simulink model "do178b_dhc2_rev_new"  (R2021b)
settings: Solver=ode23  StartTime=0.0  StopTime=25  MaxStep=1/40  RelTol=1e-2  AbsTol=1e-3  EnableMultiTasking=on
PreLoadFcn:
  | load asbdhc2_init;
  | Autopilot_bus;
model workspace (MAT data in the model file):
  ALT_Mode = [0 0 0 0 0 0 0 0 0 0 0 0 ... (1001 elements, 1001x1)]
  ALT_Ref = [991.703720962 991.703720962 991.703720962 991.703720962 991.703720962 991.703720962 991.703720962 991.703720962 991.703720962 991.703720962 991.703720962 991.703720962 ... (1001 elements, 1001x1)]
  AP_Eng = [1 1 1 1 1 1 1 1 1 1 1 1 ... (1001 elements, 1001x1)]
  AilCmdv = [0; 0; 0]
  Ail_cmd : timeseries (value not decoded)
  FR = [0; 0]
  Ft = [0 0.333333333333 0.333333333333 0.333333333333 0.333333333333 0.333333333333 0.333333333333 0.333333333333 0.333333333333 0.333333333333 0.333333333333 0.333333333333 ... (1001 elements, 1001x1)]
  HDG_Mode = [0 0 0 0 0 0 0 0 0 0 0 0 ... (1001 elements, 1001x1)]
  HDG_Ref = [29.7066688805 29.7066688805 29.7066688805 29.7066688805 29.7066688805 29.7066688805 29.7066688805 29.7066688805 29.7066688805 29.7066688805 29.7066688805 29.7066688805 ... (1001 elements, 1001x1)]
  InputSize = 2
  N = 37
  PhiRefv = [0; 0; 0]
  Phi_Ref : timeseries (value not decoded)
  Phiv = [0; 0; 0]
  Pwheel = [2.59796598511 2.59796598511 2.59796598511 2.59796598511 2.59796598511 2.59796598511 2.59796598511 2.59796598511 2.59796598511 2.59796598511 2.59796598511 2.59796598511 ... (1001 elements, 1001x1)]
  Roll_Mode = [1 1 1 1 1 1 1 1 1 1 1 1 ... (1001 elements, 1001x1)]
  TimeSteps = 1001
  Tkv = [0; 0; 0]
  TurnK = [-15.9132354515 -15.9132354515 -15.9132354515 -15.9132354515 -15.9132354515 -15.9132354515 -15.9132354515 -15.9132354515 -15.9132354515 -15.9132354515 -15.9132354515 -15.9132354515 ... (1001 elements, 1001x1)]
  X = [1 1 1 0 0 0 0 0 1 81.536789931 -1.01532751936 38.5971284353 ... (24 elements, 1x24)]
  a = 0.726747501556
  a1 = [0.30275909672 0.30275909672 0.30275909672 0.30275909672 0.30275909672 0.30275909672 0.30275909672 0.30275909672 0.30275909672 0.30275909672 0.30275909672 0.30275909672 ... (1001 elements, 1x1001)]
  apin : object (value not decoded)
  apsin : time (value not decoded)
  curPath = 'C:\Python-Workspace\thesis\new FSE2019\ModeTestingData\Problems'
  d = 25
  hws : Simulink.ModelWorkspace (value not decoded)
  i = 9
  inertial : object (value not decoded)
  j = 8
  list : object (value not decoded)
  modelpath = 'C:\Python-Workspace\thesis\new FSE2019\Benchmark\Simulink Models\autopilot\aprevised\'
  models : object (value not decoded)
  n = 1
  nbrInputs = 8
  req = 'R12.1'
  rollOut = []
  simOut : Simulink.SimulationOutput (value not decoded)
  t = [0 0.025 0.05 0.075 0.1 0.125 0.15 0.175 0.2 0.225 0.25 0.275 ... (1001 elements, 1x1001)]
undefined symbols (not defined in the file): beaver_b, beaver_c, beaver_init_p, beaver_init_pitch, beaver_init_q, beaver_init_r, beaver_init_roll, beaver_mass, Cl0, Cl_alpha2_dpt, Cl_beta, Cl_da, Cl_da_alpha, Cl_dr, Cl_p, Cl_r, Cm0, Cm_alpha, Cm_alpha2, Cm_beta2, Cm_de, Cm_df, Cm_dpt, Cm_q, Cm_r, Cn0, Cn_beta, Cn_beta3, Cn_da, Cn_dpt3, Cn_dr, Cn_p, Cn_q, Cn_r, Cx0, Cx_alpha, Cx_alpha2, Cx_alpha3, Cx_df, Cx_df_alpha, Cx_dpt, Cx_dpt2_alpha, Cx_dr, Cx_q, Cy0, Cy_beta, Cy_da, Cy_dr, Cy_dr_alpha, Cy_p, Cy_r, Cz0, Cz_alpha, Cz_alpha3, Cz_de, Cz_de_beta, Cz_df, Cz_df_alpha, Cz_dpt, Cz_q ... (+9)
libraries: aerolibconvert2 x6, simulink x6, aerolibobsolete x5, aerolibasang x3, aerolibwind2 x3, aerolibadyn x1, aerolibatmos2 x1
(part 2 of 3)

== system do178b_dhc2_rev_new/Air Data Sensor ==
  note: Air Data Sensor
  AC Bus : Inport
  Bus Creator : BusCreator  Inputs=5
  Bus Selector : BusSelector  OutputSignals=Hdot,Ve,xyh
  Length Conversion : aerolibconvert2/Length Conversion  IU=m  OU=ft
  Rate Transition1 : RateTransition  OutPortSampleTime=1/40
  Rate Transition2 : RateTransition  InitialCondition=2202  OutPortSampleTime=1/40
  Rate Transition3 : RateTransition  InitialCondition=[44.54 2.714 5.836]  OutPortSampleTime=1/40
  Selector1 : Selector  InputPortWidth=3  IndexOptions=Index vector (dialog)  Indices=[3]  OutputSizes=1
  Velocity Conversion : aerolibconvert2/Velocity Conversion  IU=m/s  OU=ft/s
  Velocity Conversion1 : aerolibconvert2/Velocity Conversion  IU=m/s  OU=ft/s
  "alpha, beta, TAS" : aerolibasang/Incidence, Sideslip, & Airspeed
  Air Data : Outport  VectorParamsAs1DForOutWhenUnconnected=off
  wires:
  AC Bus/1 -> Bus Selector/1
  Bus Selector/1 -> Velocity Conversion/1  "<Hdot>"
  Bus Selector/2 -> Rate Transition3/1  "<Ve>"
  Bus Selector/3 -> Selector1/1  "<xyh>"
  Bus Creator/1 -> Air Data/1
  Rate Transition1/1 -> Bus Creator/1  "altRate"
  Selector1/1 -> Rate Transition2/1
  "alpha, beta, TAS"/1 -> Bus Creator/2  "alpha"
  "alpha, beta, TAS"/2 -> Bus Creator/3  "beta"
  "alpha, beta, TAS"/3 -> Bus Creator/4  "airspeed"
  Velocity Conversion/1 -> Rate Transition1/1
  Length Conversion/1 -> Bus Creator/5  "alt"
  Velocity Conversion1/1 -> "alpha, beta, TAS"/1
  Rate Transition3/1 -> Velocity Conversion1/1
  Rate Transition2/1 -> Length Conversion/1

== system do178b_dhc2_rev_new/Cockpit Controls ==
  Demux : Demux  Tag=STV Demux  Outputs=2
      settings: DisplayOption=none
  FromWs : FromWorkspace  Tag=STV FromWs  VariableName=tuvar
      SigBuilderData=|
      | common.afterFinalStr = 'Extrapolate'
      | common.sampleTime = 0
      | dataSet.timeRange = [0 10]
      | dataSet.name = 'Steady State Flight'
      | sbobj.Groups.Name = 'Steady State Flight'
      | sbobj.Groups.Signals(1).Name = 'Flap Handle'
      | sbobj.Groups.Signals(1).XData = [0 10]
      | sbobj.Groups.Signals(1).YData = [0 0]
      | sbobj.Groups.Signals(2).Name = 'Rudder Trim'
      | sbobj.Groups.Signals(2).XData = [0 10]
      | sbobj.Groups.Signals(2).YData = [0 0]
  Flap Handle : Outport  Tag=STV Outport  VectorParamsAs1DForOutWhenUnconnected=off
  Rudder Trim : Outport  Tag=STV Outport  Port=2  VectorParamsAs1DForOutWhenUnconnected=off
  wires:
  FromWs/1 -> Demux/1
  Demux/1 -> Flap Handle/1
  Demux/2 -> Rudder Trim/1

== system do178b_dhc2_rev_new/DeHavilland Beaver Airframe ==
  note: DeHavilland Beaver Airframe
  EnvirBus : Inport
  Pilot : Inport  Port=2
  Aircraft Dynamics : Subsystem
  Calculate Parameters : Subsystem
  ACBus : Outport  VectorParamsAs1DForOutWhenUnconnected=off
  wires:
  Pilot/1 -> Aircraft Dynamics/1(Pilot)
  Aircraft Dynamics/1(AC Bus) -> ACBus/1, Calculate Parameters/2(ACBus)
  EnvirBus/1 -> Aircraft Dynamics/2(EnvirBus), Calculate Parameters/1(EnvirBus)
  Calculate Parameters/1(FltParams) -> Aircraft Dynamics/3(FltParams)

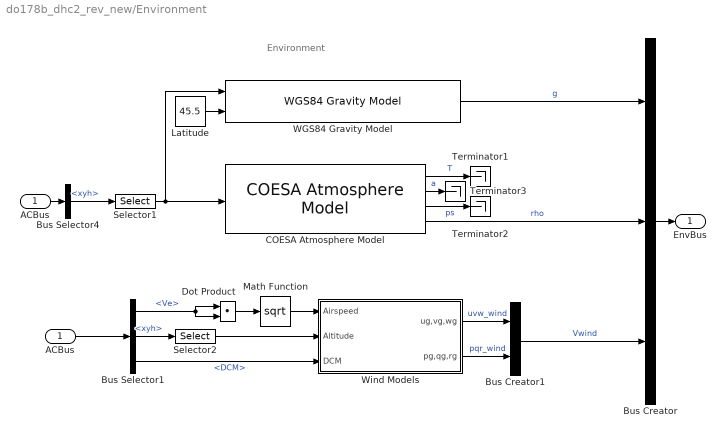
== system do178b_dhc2_rev_new/Environment ==
  note: Environment
  ACBus : Inport
  "ACBus " : InportShadow
  Bus Creator : BusCreator  Inputs=3
  Bus Creator1 : BusCreator  Inputs=2
  Bus Selector1 : BusSelector  OutputSignals=Ve,xyh,DCM
  Bus Selector4 : BusSelector  OutputSignals=xyh
  COESA Atmosphere Model : aerolibatmos2/COESA Atmosphere Model  units=Metric (MKS)  spec=1976 COESA-extended U.S. Standard Atmosphere  model=Profile  profile_var=High temperature  profile_percent=1%  profile_alt=5 km (16404 ft)  envelope_var=High temperature  envelope_percent=1%  action=Warning
  Dot Product : DotProduct  InputSameDT=on  OutDataTypeStr=Inherit: Inherit via internal rule
  Latitude : Constant  Value=45.5
  Math Function : Math  Operator=sqrt  SignedPower=on  SaturateOnIntegerOverflow=on
  Selector1 : Selector  InputPortWidth=3  IndexOptions=Index vector (dialog)  Indices=[3]  OutputSizes=1
  Selector2 : Selector  InputPortWidth=3  IndexOptions=Index vector (dialog)  Indices=[3]  OutputSizes=1
  Terminator1 : Terminator
  Terminator2 : Terminator
  Terminator3 : Terminator
  WGS84 Gravity Model : aerolibobsolete/WGS84 Gravity Model  model=WGS84 Taylor Series  units=Metric (MKS)  no_atmos=on  precessing=on  month=February  day=1  year=2000  no_centrifugal=on  action=Warning
      settings: SourceProductBaseCode=AE
  Wind Models : Subsystem
  EnvBus : Outport  VectorParamsAs1DForOutWhenUnconnected=off
  wires:
  COESA Atmosphere Model/4 -> Bus Creator/2  "rho"
  COESA Atmosphere Model/1 -> Terminator1/1  "T"
  COESA Atmosphere Model/3 -> Terminator2/1  "ps"
  COESA Atmosphere Model/2 -> Terminator3/1  "a"
  Selector1/1 -> COESA Atmosphere Model/1, WGS84 Gravity Model/1
  Latitude/1 -> WGS84 Gravity Model/2
  WGS84 Gravity Model/1 -> Bus Creator/1  "g"
  Bus Selector1/3 -> Wind Models/3(DCM)  "<DCM>"
  Wind Models/2(pg,qg,rg) -> Bus Creator1/2  "pqr_wind"
  Wind Models/1(ug,vg,wg) -> Bus Creator1/1  "uvw_wind"
  Bus Creator1/1 -> Bus Creator/3  "Vwind"
  Dot Product/1 -> Math Function/1
  Math Function/1 -> Wind Models/1(Airspeed)
  Bus Creator/1 -> EnvBus/1
  ACBus/1 -> Bus Selector4/1
  Bus Selector4/1 -> Selector1/1  "<xyh>"
  "ACBus "/1 -> Bus Selector1/1
  Bus Selector1/2 -> Selector2/1  "<xyh>"
  Selector2/1 -> Wind Models/2(Altitude)
  Bus Selector1/1 -> Dot Product/1, Dot Product/2  "<Ve>"

== system do178b_dhc2_rev_new/Inertial Data Sensor ==
  note: Inertial Data Sensor
  AC Bus : Inport
  Angle Conversion3 : aerolibconvert2/Angle Conversion  IU=rad  OU=deg
  Angle Conversion5 : aerolibconvert2/Angle Conversion  IU=rad  OU=deg
  Bus Creator : BusCreator  Inputs=6
  Bus Selector : BusSelector  OutputSignals=phi_theta_psi,pqr
  Demux : Demux  Outputs=3
  Demux1 : Demux  Outputs=3
  Rate Transition1 : RateTransition  InitialCondition=beaver_init_roll/pi*180  OutPortSampleTime=1/40
  Rate Transition2 : RateTransition  InitialCondition=beaver_init_pitch/pi*180  OutPortSampleTime=1/40
  Rate Transition3 : RateTransition  InitialCondition=heading0  OutPortSampleTime=1/40
  Rate Transition4 : RateTransition  OutPortSampleTime=1/40
  Inertial : Outport  VectorParamsAs1DForOutWhenUnconnected=off
  wires:
  AC Bus/1 -> Bus Selector/1
  Bus Selector/2 -> Angle Conversion3/1  "<pqr>"
  Demux/2 -> Bus Creator/5  "q"
  Bus Creator/1 -> Inertial/1
  Demux/3 -> Bus Creator/6  "r"
  Demux/1 -> Bus Creator/4  "p"
  Rate Transition1/1 -> Bus Creator/1  "phi"
  Rate Transition2/1 -> Bus Creator/2  "theta"
  Rate Transition3/1 -> Bus Creator/3  "psi"
  Rate Transition4/1 -> Demux/1
  Angle Conversion3/1 -> Rate Transition4/1
  Bus Selector/1 -> Angle Conversion5/1  "<phi_theta_psi>"
  Demux1/1 -> Rate Transition1/1
  Demux1/2 -> Rate Transition2/1
  Demux1/3 -> Rate Transition3/1
  Angle Conversion5/1 -> Demux1/1

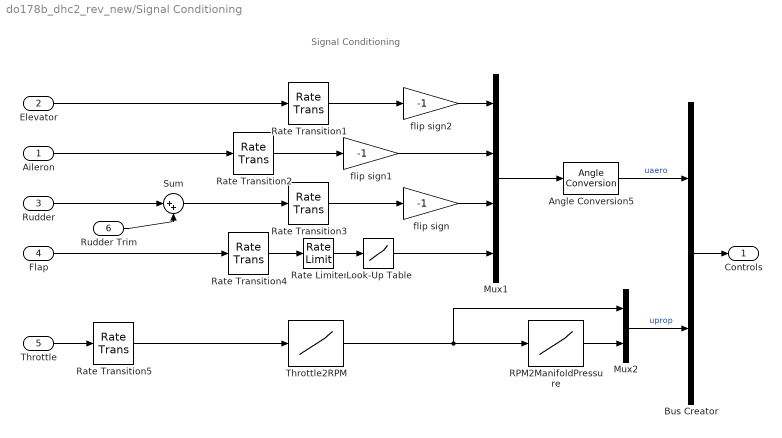
== system do178b_dhc2_rev_new/Signal Conditioning ==
  note: Signal Conditioning
  Aileron : Inport
  Elevator : Inport  Port=2
  Rudder : Inport  Port=3
  Flap : Inport  Port=4
  Throttle : Inport  Port=5
  Rudder Trim : Inport  Port=6
  Angle Conversion5 : aerolibconvert2/Angle Conversion  IU=deg  OU=rad
  Bus Creator : BusCreator  Inputs=2
  Look-Up Table : Lookup  InputValues=[0:3]  Table=[0 4 10 20]  SaturateOnIntegerOverflow=on
  Mux1 : Mux
  Mux2 : Mux  Inputs=2
  RPM2ManifoldPressure : Lookup_n-D  NumberOfTableDimensions=1  BreakpointsForDimension1=[0 1800 2300]  IndexSearchMethod=Linear search  BeginIndexSearchUsingPreviousIndexResult=on  Table=[0 22.5735 26]  ExtrapMethod=Clip  InputSameDT=on
  Rate Limiter : RateLimiter  RisingSlewLimit=0.5  FallingSlewLimit=-0.5
  Rate Transition{1..5} (5 alike) : RateTransition  OutPortSampleTime=1/40
  Sum : Sum  Inputs=|++
  Throttle2RPM : Lookup_n-D  NumberOfTableDimensions=1  BreakpointsForDimension1=(1/6)*(3+([-3:3]))  IndexSearchMethod=Linear search  BeginIndexSearchUsingPreviousIndexResult=on  Table=((1+tanh([-3:3]))/(1+tanh(2.65))-0.0025)*2300  ExtrapMethod=Clip  InputSameDT=on
  flip sign : Gain  Gain=-1  SaturateOnIntegerOverflow=on  OutDataTypeStr=Inherit: Same as input  ParamDataTypeStr=Inherit: Same as input
  flip sign1 : Gain  Gain=-1  SaturateOnIntegerOverflow=on  OutDataTypeStr=Inherit: Same as input  ParamDataTypeStr=Inherit: Same as input
  flip sign2 : Gain  Gain=-1  SaturateOnIntegerOverflow=on  OutDataTypeStr=Inherit: Same as input  ParamDataTypeStr=Inherit: Same as input
  Controls : Outport  VectorParamsAs1DForOutWhenUnconnected=off
  wires:
  Bus Creator/1 -> Controls/1
  Rate Transition5/1 -> Throttle2RPM/1
  Rate Transition4/1 -> Rate Limiter/1
  Rate Transition3/1 -> flip sign/1
  Rate Transition2/1 -> flip sign1/1
  Rate Transition1/1 -> flip sign2/1
  flip sign2/1 -> Mux1/1
  flip sign1/1 -> Mux1/2
  Throttle2RPM/1 -> RPM2ManifoldPressure/1, Mux2/1
  flip sign/1 -> Mux1/3
  Mux2/1 -> Bus Creator/2  "uprop"
  RPM2ManifoldPressure/1 -> Mux2/2
  Angle Conversion5/1 -> Bus Creator/1  "uaero"
  Mux1/1 -> Angle Conversion5/1
  Elevator/1 -> Rate Transition1/1
  Aileron/1 -> Rate Transition2/1
  Look-Up Table/1 -> Mux1/4
  Rate Limiter/1 -> Look-Up Table/1
  Flap/1 -> Rate Transition4/1
  Throttle/1 -> Rate Transition5/1
  Sum/1 -> Rate Transition3/1
  Rudder/1 -> Sum/1
  Rudder Trim/1 -> Sum/2

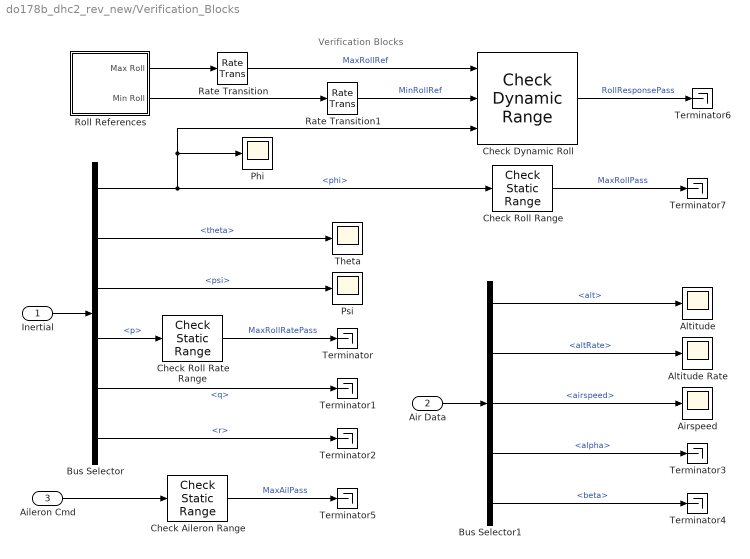
== system do178b_dhc2_rev_new/Verification_Blocks ==
  note: Verification Blocks
  Inertial : Inport
  Air Data : Inport  Port=2
  Aileron Cmd : Inport  Port=3
  Airspeed : Scope
  Altitude : Scope
  Altitude Rate : Scope
  Bus Selector : BusSelector  OutputSignals=phi,theta,psi,p,q,r
  Bus Selector1 : BusSelector  OutputSignals=alt,altRate,airspeed,alpha,beta
  Check Aileron Range : simulink/Model Verification/Check  Static Range  Description=-15 <= u <= 15  max=15  max_included=on  min=-15  min_included=on  enabled=on  stopWhenAssertionFail=off  export=on  icon=graphic
      settings: AttributesFormatString=%<Description>  SourceProductBaseCode=SL
  Check Dynamic Roll : simulink/Model Verification/Check  Dynamic Range  Description=min < u < max  enabled=on  stopWhenAssertionFail=off  export=on  icon=graphic
      settings: SourceProductBaseCode=SL
  Check Roll Range : simulink/Model Verification/Check  Static Range  Description=-33 <= u <= 33  max=33  max_included=on  min=-33  min_included=on  enabled=on  stopWhenAssertionFail=off  export=on  icon=graphic
      settings: AttributesFormatString=%<Description>  SourceProductBaseCode=SL
  Check Roll Rate Range : simulink/Model Verification/Check  Static Range  Description=-6.6 <= u <= 6.6  max=6.6  max_included=on  min=-6.6  min_included=on  enabled=on  stopWhenAssertionFail=off  export=on  icon=graphic
      settings: AttributesFormatString=%<Description>  SourceProductBaseCode=SL
  Phi : Scope
  Psi : Scope
  Rate Transition : RateTransition  InitialCondition=beaver_init_roll/pi*180+1  OutPortSampleTime=1/40
  Rate Transition1 : RateTransition  InitialCondition=beaver_init_roll/pi*180-1  OutPortSampleTime=1/40
  Roll References : Subsystem  Tag=STV Subsys  RequirementInfo={'other' 'do178b_autopilot_requirements.doc' '1.1. Roll Autopilot Engage Control' 'true' '1.1. Roll Autopilot Engage Control' '' ; 'other' 'do178b_autopilot_requirements.doc' '@1.2. Roll Hold Mode' 'true' '1.2. Roll Hold Mode' ' ' ; 'other' 'do178b_autopilot_requirements.doc' '@1.3. Roll Hold Reference' 'true' '1.3. Roll Hold Reference' ' ' ; 'other' 'do178b_autopilot_requirements.doc' '1.1. Roll Autopilot Engage Control' 'true' '1.1. Roll Autopilot Engage Control' '' ; 'other' 'do178b_autopilot_requirements.doc' '1.2. Roll Hold Mode' 'true' '1.2. Roll Hold Mode' '' ; 'other' 'do178b_autopilot_requirements.doc' '1.3. Roll Hold Reference' 'true' '1.3. Roll Hold Reference' '' ; 'other' 'do178b_autopilot_requirements.doc' '1.1. Roll Autopilot Engage Control' 'true' '1.1. Roll Autopilot Engage Control' '' ; 'other' 'do178b_autopilot_requirements.doc' '1.2. Roll Hold Mode' 'true' '1.2. Roll Hold Mode' '' ; 'other' 'do178b_autopilot_requirements.doc' '1.3. Roll Hold Reference' 'true' '1.3. Roll Hold Reference' '' ; 'other' 'do178b_autopilot_requirements.doc' '1.1. Roll Autopilot Engage Control' 'true' '1.1. Roll Autopilot Engage Control' '' ; 'other' 'do178b_autopilot_requirements.doc' '1.2. Roll Hold Mode' 'true' '1.2. Roll Hold Mode' '' ; 'other' 'do178b_autopilot_requirements.doc' '1.3. Roll Hold Reference' 'true' '1.3. Roll Hold Reference' '' ; 'other' 'do178b_autopilot_requirements.doc' '1.1. Roll Autopilot Engage Control' 'true' '1.1. Roll Autopilot Engage Control' '' ; 'other' 'do178b_autopilot_requirements.doc' '1.2. Roll Hold Mode' 'true' '1.2. Roll Hold Mode' '' ; 'other' 'do178b_autopilot_requirements.doc' '1.3. Roll Hold Reference' 'true' '1.3. Roll Hold Reference' '' ; 'other' 'do178b_autopilot_requirements.doc' '1.1. Roll Autopilot Engage Control' 'true' '1.1. Roll Autopilot Engage Control' '' ; 'other' 'do178b_autopilot_requirements.doc' '1.2. Roll Hold Mode' 'true' '1.2. Roll Hold Mode' '' ; 'other' 'do178b_autopilot_requirements.doc' '1.3. Roll Hold Reference' 'true' '1.3. Roll Hold Reference' '' ; 'other' 'do178b_autopilot_requirements.doc' '1.1. Roll Autopilot Engage Control' 'true' '1.1. Roll Autopilot Engage Control' '' ; 'other' 'do178b_autopilot_requirements.doc' '1.2. Roll Hold Mode' 'true' '1.2. Roll Hold Mode' '' ; 'other' 'do178b_autopilot_requirements.doc' '1.3. Roll Hold Reference' 'true' '1.3. Roll Hold Reference' '' ; 'other' 'do178b_autopilot_requirements.doc' '1.1. Roll Autopilot Engage Control' 'true' '1.1. Roll Autopilot Engage Control' '' ; 'other' 'do178b_autopilot_requirements.doc' '1.2. Roll Hold Mode' 'true' '1.2. Roll Hold Mode' '' ; 'other' 'do178b_autopilot_requirements.doc' '1.3. Roll Hold Reference' 'true' '1.3. Roll Hold Reference' '' ; 'other' 'do178b_autopilot_requirements.doc' '1.1. Roll Autopilot Engage Control' 'true' '1.1. Roll Autopilot Engage Control' '' ; 'other' 'do178b_autopilot_requirements.doc' '1.2. Roll Hold Mode' 'true' '1.2. Roll Hold Mode' '' ; 'other' 'do178b_autopilot_requirements.doc' '1.3. Roll Hold Reference' 'true' '1.3. Roll Hold Reference' '' ; 'other' 'do178b_autopilot_requirements.doc' '1.1. Roll Autopilot Engage Control' 'true' '1.1. Roll Autopilot Engage Control' '' ; 'other' 'do178b_autopilot_requirements.doc' '1.2. Roll Hold Mode' 'true' '1.2. Roll Hold Mode' '' ; 'other' 'do178b_autopilot_requirements.doc' '1.3. Roll Hold Reference' 'true' '1.3. Roll Hold Reference' '' ; 'other' 'do178b_autopilot_requirements.doc' '1.1. Roll Autopilot Engage Control' 'true' '1.1. Roll Autopilot Engage Control' '' ; 'other' 'do178b_autopilot_requirements.doc' '1.2. Roll Hold Mode' 'true' '1.2. Roll Hold Mode' '' ; 'other' 'do178b_autopilot_requirements.doc' '1.3. Roll Hold Reference' 'true' '1.3. Roll Hold Reference' '' ; 'other' 'do178b_autopilot_requirements.doc' '1.1. Roll Autopilot Engage Control' 'true' '1.1. Roll Autopilot Engage Control' '' ; 'other' 'do178b_autopilot_requirements.doc' '1.2. Roll Hold Mode' 'true' '1.2. Roll Hold Mode' '' ; 'other' 'do178b_autopilot_requirements.doc' '1.3. Roll Hold Reference' 'true' '1.3. Roll Hold Reference' '' ; 'other' 'do178b_autopilot_requirements.doc' '1.1. Roll Autopilot Engage Control' 'true' '1.1. Roll Autopilot Engage Control' '' ; 'other' 'do178b_autopilot_requirements.doc' '1.2. Roll Hold Mode' 'true' '1.2. Roll Hold Mode' '' ; 'other' 'do178b_autopilot_requirements.doc' '1.3. Roll Hold Reference' 'true' '1.3. Roll Hold Reference' '' ; 'other' 'do178b_autopilot_requirements.doc' '1.1. Roll Autopilot Engage Control' 'true' '1.1. Roll Autopilot Engage Control' '' ; 'other' 'do178b_autopilot_requirements.doc' '1.2. Roll Hold Mode' 'true' '1.2. Roll Hold Mode' '' ; 'other' 'do178b_autopilot_requirements.doc' '1.3. Roll Hold Reference' 'true' '1.3. Roll Hold Reference' '' ; 'other' 'do178b_autopilot_requirements.doc' '1.1. Roll Autopilot Engage Control' 'true' '1.1. Roll Autopilot Engage Control' '' ; 'other' 'do178b_autopilot_requirements.doc' '1.2. Roll Hold Mode' 'true' '1.2. Roll Hold Mode' '' ; 'other' 'do178b_autopilot_requirements.doc' '1.3. Roll Hold Reference' 'true' '1.3. Roll Hold Reference' '' ; 'other' 'do178b_autopilot_requirements.doc' '1.1. Roll Autopilot Engage Control' 'true' '1.1. Roll Autopilot Engage Control' '' ; 'other' 'do178b_autopilot_requirements.doc' '1.2. Roll Hold Mode' 'true' '1.2. Roll Hold Mode' '' ; 'other' 'do178b_autopilot_requirements.doc' '1.3. Roll Hold Reference' 'true' '1.3. Roll Hold Reference' '' ; 'other' 'do178b_autopilot_requirements.doc' '1.4. Roll Performance' 'true' '1.4. Roll Performance' '' ; 'other' 'do178b_autopilot_requirements.doc' '1.4. Roll Performance' 'true' '1.4. Roll Performance' '' ; 'other' 'do178b_autopilot_requirements.doc' '1.5. Roll Rate Limit' 'true' '1.5. Roll Rate Limit' '' ; 'other' 'do178b_autopilot_requirements.doc' '1.6. Roll Angle Limit' 'true' '1.6. Roll Angle Limit' '' ; 'other' 'do178b_autopilot_requirements.doc' '1.7. Aileron Angle Limit' 'true' '1.7. Aileron Angle Limit' '' ; 'other' 'do178b_autopilot_requirements.doc' '@1.5. Roll Rate Limit' 'true' '1.5. Roll Rate Limit' ' ' ; 'other' 'do178b_autopilot_requirements.doc' '@1.6. Roll Angle Limit' 'true' '1.6. Roll Angle Limit' ' ' ; 'other' 'do178b_autopilot_requirements.doc' '1.7. Aileron Angle Limit' 'true' '1.7. Aileron Angle Limit' '' } %GIDa_ba1e5288_f274_4b44_a12a_943497d6d101  LoadFcn=sigbuilder_block('load');  StartFcn=sigbuilder_block('start');  StopFcn=sigbuilder_block('stop');  ClipboardFcn=sigbuilder_block('clipboard');  mask(Sigbuilder block){tuvar=[0:10]}
      mask help: Sigbuilder GUI
      mask init:
      | if ~strcmp(get_param(bdroot(gcbh),'SimulationStatus'),'stopped') tuvar = sigbuilder_block('maskInit'); end
      settings: CopyFcn=sigbuilder_block('copy');  DeleteFcn=sigbuilder_block('delete');  ModelCloseFcn=sigbuilder_block('modelClose');  PreSaveFcn=sigbuilder_block('preSave');  PauseFcn=sigbuilder_block('pause')  ContinueFcn=sigbuilder_block('continue')  NameChangeFcn=sigbuilder_block('namechange');  OpenFcn=sigbuilder_block('open',[588 171 707 381 ]);  CloseFcn=sigbuilder_block('close');
      mask Display: plot(0, 0, 100, 100,[2, 2, 32, 32, 2], [68, 8, 8, 68, 68],[32, 2], [38, 38], [32, 19, 2],[53, 60, 44], [32, 17, 17, 2],[16, 16, 31, 31]);txt = getActiveGroup(gcbh);text(2, 100, txt,'verticalAlignment', 'top');
  Terminator{,1..7} (8 alike) : Terminator
  Theta : Scope
  wires:
  Inertial/1 -> Bus Selector/1
  Bus Selector/1 -> Check Roll Range/1, Check Dynamic Roll/3, Phi/1  "<phi>"
  Bus Selector/2 -> Theta/1  "<theta>"
  Bus Selector/3 -> Psi/1  "<psi>"
  Bus Selector/4 -> Check Roll Rate Range/1  "<p>"
  Bus Selector/5 -> Terminator1/1  "<q>"
  Bus Selector/6 -> Terminator2/1  "<r>"
  Bus Selector1/1 -> Altitude/1  "<alt>"
  Bus Selector1/2 -> Altitude Rate/1  "<altRate>"
  Bus Selector1/3 -> Airspeed/1  "<airspeed>"
  Bus Selector1/4 -> Terminator3/1  "<alpha>"
  Bus Selector1/5 -> Terminator4/1  "<beta>"
  Aileron Cmd/1 -> Check Aileron Range/1
  Check Aileron Range/1 -> Terminator5/1  "MaxAilPass"
  Check Roll Rate Range/1 -> Terminator/1  "MaxRollRatePass"
  Check Dynamic Roll/1 -> Terminator6/1  "RollResponsePass"
  Roll References/1(Max Roll) -> Rate Transition/1
  Roll References/2(Min Roll) -> Rate Transition1/1
  Check Roll Range/1 -> Terminator7/1  "MaxRollPass"
  Rate Transition/1 -> Check Dynamic Roll/1  "MaxRollRef"
  Rate Transition1/1 -> Check Dynamic Roll/2  "MinRollRef"
  Air Data/1 -> Bus Selector1/1

== system do178b_dhc2_rev_new/DeHavilland Beaver Airframe/Aircraft Dynamics ==
  Pilot : Inport
  EnvirBus : Inport  Port=2
  FltParams : Inport  Port=3
  6DoF (Quaternion) : aerolibobsolete/6DoF (Euler Angles)  units=Metric (MKS)  mtype=Fixed  rep=Quaternion  xme_0=xme_0  Vm_0=[44.54 2.714 5.836]  eul_0=[beaver_init_roll, beaver_init_pitch, heading0/180*pi]  pm_0=[beaver_init_p, beaver_init_q, beaver_init_r]  mass_0=beaver_mass  mass_e=0  mass_f=0  inertia="[5.787969e3  0 1.1764e2; 0 6.92893e3 0; -1.1764e2 0 1.1578329e4]"  inertia_e=eye(3)  inertia_f=eye(3)  k_quat=1.0
      settings: SourceProductBaseCode=AE
  Bus Creator : BusCreator  Inputs=8
  Hdot : Gain  Gain=-1  SaturateOnIntegerOverflow=on  OutDataTypeStr=Inherit: Same as input  ParamDataTypeStr=Inherit: Same as input
  Selector1 : Selector  InputPortWidth=3  IndexOptions=Index vector (dialog)  Indices=[3]  OutputSizes=1
  Terminator : Terminator
  Terminator1 : Terminator
  Total Forces and Moments : Subsystem
  xyH : Gain  Gain=[1 1 -1]  SaturateOnIntegerOverflow=on  OutDataTypeStr=Inherit: Same as input  ParamDataTypeStr=Inherit: Same as input
  AC Bus : Outport  VectorParamsAs1DForOutWhenUnconnected=off
  wires:
  6DoF (Quaternion)/4 -> Bus Creator/6, Total Forces and Moments/3(DCM)  "DCM"
  6DoF (Quaternion)/3 -> Bus Creator/5  "phi_theta_psi"
  6DoF (Quaternion)/2 -> xyH/1, Bus Creator/3  "Xe"
  6DoF (Quaternion)/5 -> Bus Creator/7  "Vbody"
  6DoF (Quaternion)/7 -> Terminator/1
  6DoF (Quaternion)/1 -> Selector1/1, Bus Creator/2  "Ve"
  Pilot/1 -> Total Forces and Moments/2(Pilot)
  Selector1/1 -> Hdot/1
  Total Forces and Moments/1(Total Force) -> 6DoF (Quaternion)/1
  Total Forces and Moments/2(Total Moment) -> 6DoF (Quaternion)/2
  xyH/1 -> Bus Creator/4  "xyh"
  Hdot/1 -> Bus Creator/1  "Hdot"
  6DoF (Quaternion)/8 -> Terminator1/1
  Bus Creator/1 -> AC Bus/1
  EnvirBus/1 -> Total Forces and Moments/1(EnvirBus)
  6DoF (Quaternion)/6 -> Bus Creator/8  "pqr"
  FltParams/1 -> Total Forces and Moments/4(FltParams)

== system do178b_dhc2_rev_new/DeHavilland Beaver Airframe/Calculate Parameters ==
  EnvirBus : Inport
  ACBus : Inport  Port=2
  "ACBus " : InportShadow  Port=2
  Bus Creator : BusCreator  Inputs=5
  Bus Selector1 : BusSelector  OutputSignals=rho
  Bus Selector2 : BusSelector  OutputSignals=Vbody
  Bus Selector3 : BusSelector  OutputSignals=pqr,Ve
  Bus Selector4 : BusSelector  OutputSignals=Vwind.uvw_wind,Vwind.pqr_wind
  Dynamic Pressure : aerolibasang/Dynamic Pressure
  "Incidence, Sideslip, & Airspeed" : aerolibasang/Incidence, Sideslip, & Airspeed
  Sum2 : Sum  Inputs=|++  InputSameDT=on  SaturateOnIntegerOverflow=on  OutDataTypeStr=Inherit: Same as first input
  Sum4 : Sum  Inputs=+-|  InputSameDT=on  SaturateOnIntegerOverflow=on  OutDataTypeStr=Inherit: Same as first input
  FltParams : Outport  VectorParamsAs1DForOutWhenUnconnected=off
  wires:
  "ACBus "/1 -> Bus Selector2/1
  Bus Creator/1 -> FltParams/1
  Bus Selector3/1 -> Sum2/2  "<pqr>"
  ACBus/1 -> Bus Selector3/1
  Bus Selector1/1 -> Dynamic Pressure/2  "<rho>"
  EnvirBus/1 -> Bus Selector1/1, Bus Selector4/1
  Dynamic Pressure/1 -> Bus Creator/5  "Qdyn"
  Bus Selector3/2 -> Dynamic Pressure/1  "<Ve>"
  Bus Selector4/2 -> Sum2/1  "<pqr_wind>"
  Sum4/1 -> "Incidence, Sideslip, & Airspeed"/1
  "Incidence, Sideslip, & Airspeed"/1 -> Bus Creator/1  "alpha"
  "Incidence, Sideslip, & Airspeed"/2 -> Bus Creator/2  "beta"
  "Incidence, Sideslip, & Airspeed"/3 -> Bus Creator/3  "V"
  Bus Selector2/1 -> Sum4/1  "<Vbody>"
  Bus Selector4/1 -> Sum4/2  "<uvw_wind>"
  Sum2/1 -> Bus Creator/4  "pqr_tot"

== system do178b_dhc2_rev_new/Environment/Wind Models ==
  Airspeed : Inport
  Altitude : Inport  Port=2
  DCM : Inport  Port=3
  "DCM " : InportShadow  Port=3
  Discrete Wind Gust Model : aerolibwind2/Discrete Wind Gust Model  units=Metric (MKS)  Gx=off  Gy=off  Gz=off  t_0=20  d_m=[120 120 80]  v_m=[3.5 3.5 3.0]
  Dryden Wind Turbulence Model (Continuous (+q -r)) : aerolibwind2/Dryden Wind Turbulence Model  (Continuous (+q -r))  units=Metric (MKS)  spec=MIL-F-8785C  model=Continuous Dryden (+q -r)  W20=5  Wdeg=0  TurbProb=10^-2 - Light  L_high=533.4  Wingspan=4  ts=0.1  Seed=[23341 23342 23343 23344]  T_on=off
  Sum : Sum  Inputs=+++  InputSameDT=on  SaturateOnIntegerOverflow=on  OutDataTypeStr=Inherit: Same as first input
  Wind Shear Model : aerolibwind2/Wind Shear Model  units=Metric (MKS)  phase=Category C - Terminal Flight Phase  W_20=0  Wdeg=0
  ug,vg,wg : Outport  VectorParamsAs1DForOutWhenUnconnected=off
  pg,qg,rg : Outport  Port=2  VectorParamsAs1DForOutWhenUnconnected=off
  wires:
  "DCM "/1 -> Dryden Wind Turbulence Model (Continuous (+q -r))/3
  Wind Shear Model/1 -> Sum/1
  Dryden Wind Turbulence Model (Continuous (+q -r))/1 -> Sum/2
  Discrete Wind Gust Model/1 -> Sum/3
  Sum/1 -> ug,vg,wg/1
  DCM/1 -> Wind Shear Model/2
  Airspeed/1 -> Dryden Wind Turbulence Model (Continuous (+q -r))/2, Discrete Wind Gust Model/1
  Dryden Wind Turbulence Model (Continuous (+q -r))/2 -> pg,qg,rg/1
  Altitude/1 -> Dryden Wind Turbulence Model (Continuous (+q -r))/1, Wind Shear Model/1

== system do178b_dhc2_rev_new/Verification_Blocks/Roll References ==
  Demux : Demux  Tag=STV Demux  Outputs=2
      settings: DisplayOption=none
  FromWs : FromWorkspace  Tag=STV FromWs  VariableName=tuvar
      SigBuilderData=|
      | common.afterFinalStr = 'Extrapolate'
      | common.sampleTime = 0
      | dataSet(1).timeRange = [0 25]
      | dataSet(1).name = 'Roll Test 1'
      | dataSet(2).timeRange = [0 25]
      | dataSet(2).name = 'Roll Test 2'
      | dataSet(3).timeRange = [0 25]
      | dataSet(3).name = 'Roll Test 3'
      | dataSet(4).timeRange = [0 25]
      | dataSet(4).name = 'Roll Test 4'
      | dataSet(5).timeRange = [0 25]
      | dataSet(5).name = 'Roll Test 5'
      | dataSet(6).timeRange = [0 25]
      | dataSet(6).name = 'Roll Test 6'
      | dataSet(7).timeRange = [0 25]
      | dataSet(7).name = 'Roll Test 7'
      | dataSet(8).timeRange = [0 25]
      | dataSet(8).name = 'Roll Test 8'
      | dataSet(9).timeRange = [0 25]
      | dataSet(9).name = 'Roll Test 9'
      | dataSet(10).timeRange = [0 25]
      | dataSet(10).name = 'Roll Test 10'
      | dataSet(11).timeRange = [0 25]
      | dataSet(11).name = 'Roll Test 11'
      | dataSet(12).timeRange = [0 25]
      | dataSet(12).name = 'Roll Test 12'
      | dataSet(13).timeRange = [0 25]
      | dataSet(13).name = 'Roll Test 13'
      | dataSet(14).timeRange = [0 25]
      | dataSet(14).name = 'Roll Test 14'
      | dataSet(15).timeRange = [0 25]
      | dataSet(15).name = 'Roll Test 15'
      | dataSet(16).timeRange = [0 25]
      | dataSet(16).name = 'Roll Test 16'
      | dataSet(17).timeRange = [0 25]
      | dataSet(17).name = 'Roll Test 17'
      | dataSet(18).timeRange = [0 25]
      | dataSet(18).name = 'Roll Test 18'
      | dataSet(19).timeRange = [0 25]
      | dataSet(19).name = 'Roll Test 19'
      | dataSet(20).timeRange = [0 25]
      | dataSet(20).name = 'Roll Test 20'
      | sbobj.Groups(1).Name = 'Roll Test 1'
      | sbobj.Groups(1).Signals(1).Name = 'Max Roll'
      | sbobj.Groups(1).Signals(1).XData = [0 25]
      | sbobj.Groups(1).Signals(1).YData = [1 1]
      | sbobj.Groups(1).Signals(2).Name = 'Min Roll'
      | sbobj.Groups(1).Signals(2).XData = [0 25]
      | sbobj.Groups(1).Signals(2).YData = [-1 -1]
      | sbobj.Groups(2).Name = 'Roll Test 2'
      | sbobj.Groups(2).Signals(1).Name = 'Max Roll'
      | sbobj.Groups(2).Signals(1).XData = [0 2.1 2.1 6.1 6.1 25]
      | sbobj.Groups(2).Signals(1).YData = [4.1 4.1 1.6 1.6 1 1]
      | sbobj.Groups(2).Signals(2).Name = 'Min Roll'
      | sbobj.Groups(2).Signals(2).XData = [0 25]
      | sbobj.Groups(2).Signals(2).YData = [-1 -1]
      | sbobj.Groups(3).Name = 'Roll Test 3'
      | sbobj.Groups(3).Signals(1).Name = 'Max Roll'
      | sbobj.Groups(3).Signals(1).XData = [0 25]
      | sbobj.Groups(3).Signals(1).YData = [1 1]
      | sbobj.Groups(3).Signals(2).Name = 'Min Roll'
      | sbobj.Groups(3).Signals(2).XData = [0 2.1 2.1 6.1 6.1 25]
      | sbobj.Groups(3).Signals(2).YData = [-4.1 -4.1 -1.6 -1.6 -1 -1]
      | sbobj.Groups(4).Name = 'Roll Test 4'
      | sbobj.Groups(4).Signals(1).Name = 'Max Roll'
      | sbobj.Groups(4).Signals(1).XData = [0 25]
      | sbobj.Groups(4).Signals(1).YData = [9 9]
      | sbobj.Groups(4).Signals(2).Name = 'Min Roll'
      | sbobj.Groups(4).Signals(2).XData = [0 25]
      | sbobj.Groups(4).Signals(2).YData = [7 7]
      | sbobj.Groups(5).Name = 'Roll Test 5'
      | sbobj.Groups(5).Signals(1).Name = 'Max Roll'
      | sbobj.Groups(5).Signals(1).XData = [0 25]
      | sbobj.Groups(5).Signals(1).YData = [-7 -7]
      | sbobj.Groups(5).Signals(2).Name = 'Min Roll'
      | sbobj.Groups(5).Signals(2).XData = [0 25]
      | sbobj.Groups(5).Signals(2).YData = [-9 -9]
      | sbobj.Groups(6).Name = 'Roll Test 6'
      | sbobj.Groups(6).Signals(1).Name = 'Max Roll'
      | sbobj.Groups(6).Signals(1).XData = [0 25]
      | sbobj.Groups(6).Signals(1).YData = [29 29]
      | sbobj.Groups(6).Signals(2).Name = 'Min Roll'
      | sbobj.Groups(6).Signals(2).XData = [0 25]
      | sbobj.Groups(6).Signals(2).YData = [27 27]
      | sbobj.Groups(7).Name = 'Roll Test 7'
      | sbobj.Groups(7).Signals(1).Name = 'Max Roll'
      | sbobj.Groups(7).Signals(1).XData = [0 25]
      | sbobj.Groups(7).Signals(1).YData = [-27 -27]
      | sbobj.Groups(7).Signals(2).Name = 'Min Roll'
      | sbobj.Groups(7).Signals(2).XData = [0 25]
      | sbobj.Groups(7).Signals(2).YData = [-29 -29]
      | sbobj.Groups(8).Name = 'Roll Test 8'
      | sbobj.Groups(8).Signals(1).Name = 'Max Roll'
      | sbobj.Groups(8).Signals(1).XData = [0 6.1 6.1 25]
      | sbobj.Groups(8).Signals(1).YData = [32.1 32.1 31 31]
      | sbobj.Groups(8).Signals(2).Name = 'Min Roll'
      | sbobj.Groups(8).Signals(2).XData = [0 25]
      | sbobj.Groups(8).Signals(2).YData = [29 29]
      | sbobj.Groups(9).Name = 'Roll Test 9'
      | sbobj.Groups(9).Signals(1).Name = 'Max Roll'
      | sbobj.Groups(9).Signals(1).XData = [0 25]
      | sbobj.Groups(9).Signals(1).YData = [-29 -29]
      | sbobj.Groups(9).Signals(2).Name = 'Min Roll'
      | sbobj.Groups(9).Signals(2).XData = [0 6.1 6.1 25]
      | sbobj.Groups(9).Signals(2).YData = [-32.1 -32.1 -31 -31]
      | sbobj.Groups(10).Name = 'Roll Test 10'
      | sbobj.Groups(10).Signals(1).Name = 'Max Roll'
      | sbobj.Groups(10).Signals(1).XData = [0 25]
      | sbobj.Groups(10).Signals(1).YData = [1 1]
      | sbobj.Groups(10).Signals(2).Name = 'Min Roll'
      | sbobj.Groups(10).Signals(2).XData = [0 25]
      | sbobj.Groups(10).Signals(2).YData = [-1 -1]
      | sbobj.Groups(11).Name = 'Roll Test 11'
      | sbobj.Groups(11).Signals(1).Name = 'Max Roll'
      | sbobj.Groups(11).Signals(1).XData = [0 25]
      | sbobj.Groups(11).Signals(1).YData = [1 1]
      | sbobj.Groups(11).Signals(2).Name = 'Min Roll'
      | sbobj.Groups(11).Signals(2).XData = [0 25]
      | sbobj.Groups(11).Signals(2).YData = [-1 -1]
      | sbobj.Groups(12).Name = 'Roll Test 12'
      | sbobj.Groups(12).Signals(1).Name = 'Max Roll'
      | sbobj.Groups(12).Signals(1).XData = [0 25]
      | sbobj.Groups(12).Signals(1).YData = [1 1]
      | sbobj.Groups(12).Signals(2).Name = 'Min Roll'
      | sbobj.Groups(12).Signals(2).XData = [0 25]
      | sbobj.Groups(12).Signals(2).YData = [-1 -1]
      | sbobj.Groups(13).Name = 'Roll Test 13'
      | sbobj.Groups(13).Signals(1).Name = 'Max Roll'
      | sbobj.Groups(13).Signals(1).XData = [0 0.1 0.6 4 4 25]
      | sbobj.Groups(13).Signals(1).YData = [0.95 1 5 5.05 5 5]
      | sbobj.Groups(13).Signals(2).Name = 'Min Roll'
      | sbobj.Groups(13).Signals(2).XData = [0 6.1 6.1 25]
      | sbobj.Groups(13).Signals(2).YData = [-1 -1 3 3]
      | sbobj.Groups(14).Name = 'Roll Test 14'
      | sbobj.Groups(14).Signals(1).Name = 'Max Roll'
      | sbobj.Groups(14).Signals(1).XData = [0 6.1 6.1 25]
      | sbobj.Groups(14).Signals(1).YData = [1 1 -3 -3]
      | sbobj.Groups(14).Signals(2).Name = 'Min Roll'
      | sbobj.Groups(14).Signals(2).XData = [0 0.1 0.6 25]
      | sbobj.Groups(14).Signals(2).YData = [-1 -1 -5 -5]
      | sbobj.Groups(15).Name = 'Roll Test 15'
      | sbobj.Groups(15).Signals(1).Name = 'Max Roll'
      | sbobj.Groups(15).Signals(1).XData = [0 0.1 4.5 25]
      | sbobj.Groups(15).Signals(1).YData = [1 1 31 31]
      | sbobj.Groups(15).Signals(2).Name = 'Min Roll'
      | sbobj.Groups(15).Signals(2).XData = [0 2.1 9.6 25]
      | sbobj.Groups(15).Signals(2).YData = [-1 -1 29 29]
      | sbobj.Groups(16).Name = 'Roll Test 16'
      | sbobj.Groups(16).Signals(1).Name = 'Max Roll'
      | sbobj.Groups(16).Signals(1).XData = [0 2.1 9.6 25]
      | sbobj.Groups(16).Signals(1).YData = [1 1 -29 -29]
      | sbobj.Groups(16).Signals(2).Name = 'Min Roll'
      | sbobj.Groups(16).Signals(2).XData = [0 0.1 0.6 4.5 25]
      | sbobj.Groups(16).Signals(2).YData = [-1 -1 -4 -31 -31]
      | sbobj.Groups(17).Name = 'Roll Test 17'
      | sbobj.Groups(17).Signals(1).Name = 'Max Roll'
      | sbobj.Groups(17).Signals(1).XData = [0 10 10 25]
      | sbobj.Groups(17).Signals(1).YData = [1 1 4 4]
      | sbobj.Groups(17).Signals(2).Name = 'Min Roll'
      | sbobj.Groups(17).Signals(2).XData = [0 12 12 14 14 25]
      | sbobj.Groups(17).Signals(2).YData = [-1 -1 1.6 1.6 2 2]
      | sbobj.Groups(18).Name = 'Roll Test 18'
      | sbobj.Groups(18).Signals(1).Name = 'Max Roll'
      | sbobj.Groups(18).Signals(1).XData = [0 12 12 14 14 25]
      | sbobj.Groups(18).Signals(1).YData = [1 1 -1.6 -1.6 -2 -2]
      | sbobj.Groups(18).Signals(2).Name = 'Min Roll'
      | sbobj.Groups(18).Signals(2).XData = [0 10 10 25]
      | sbobj.Groups(18).Signals(2).YData = [-1 -1 -4 -4]
      | sbobj.Groups(19).Name = 'Roll Test 19'
      | sbobj.Groups(19).Signals(1).Name = 'Max Roll'
      | sbobj.Groups(19).Signals(1).XData = [0 10 15 25]
      | sbobj.Groups(19).Signals(1).YData = [1 1 33 33]
      | sbobj.Groups(19).Signals(2).Name = 'Min Roll'
      | sbobj.Groups(19).Signals(2).XData = [0 12 19 25]
      | sbobj.Groups(19).Signals(2).YData = [-1 -1 29 29]
      | sbobj.Groups(20).Name = 'Roll Test 20'
      | sbobj.Groups(20).Signals(1).Name = 'Max Roll'
      | sbobj.Groups(20).Signals(1).XData = [0 12 19 25]
      | sbobj.Groups(20).Signals(1).YData = [1 1 -29 -29]
      | sbobj.Groups(20).Signals(2).Name = 'Min Roll'
      | sbobj.Groups(20).Signals(2).XData = [0 10 15 25]
      | sbobj.Groups(20).Signals(2).YData = [-1 -1 -33 -33]
  Max Roll : Outport  Tag=STV Outport  VectorParamsAs1DForOutWhenUnconnected=off
  Min Roll : Outport  Tag=STV Outport  Port=2  VectorParamsAs1DForOutWhenUnconnected=off
  wires:
  Demux/1 -> Max Roll/1
  FromWs/1 -> Demux/1
  Demux/2 -> Min Roll/1

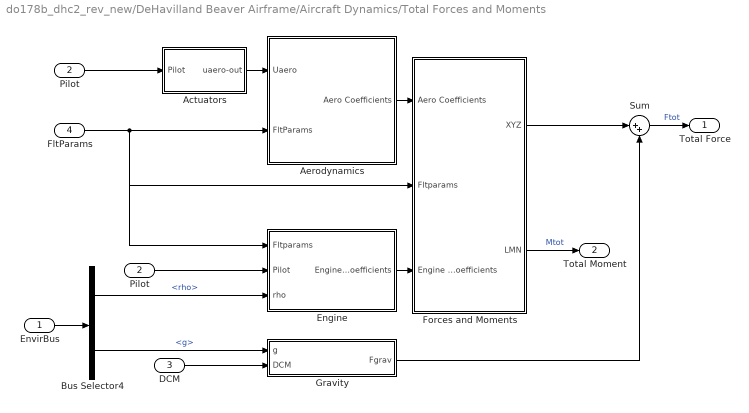
== system do178b_dhc2_rev_new/DeHavilland Beaver Airframe/Aircraft Dynamics/Total Forces and Moments ==
  EnvirBus : Inport
  Pilot : Inport  Port=2
  DCM : Inport  Port=3
  FltParams : Inport  Port=4
  Actuators : Subsystem
  Aerodynamics : Subsystem
  Bus Selector4 : BusSelector  OutputSignals=rho,g
  "Engine " : Subsystem
  Forces and Moments : Subsystem
  "Gravity " : Subsystem
  "Pilot " : InportShadow  Port=2
  Sum : Sum  Inputs=|++  InputSameDT=on  SaturateOnIntegerOverflow=on  OutDataTypeStr=Inherit: Same as first input
  Total Force : Outport  VectorParamsAs1DForOutWhenUnconnected=off
  Total Moment : Outport  Port=2  VectorParamsAs1DForOutWhenUnconnected=off
  wires:
  Forces and Moments/1(XYZ) -> Sum/1
  "Engine "/1(Engine Coefficients) -> Forces and Moments/3(Engine Coefficients)
  "Gravity "/1(Fgrav) -> Sum/2
  Aerodynamics/1(Aero Coefficients) -> Forces and Moments/1(Aero Coefficients)
  Pilot/1 -> Actuators/1(Pilot)
  Bus Selector4/1 -> "Engine "/3(rho)  "<rho>"
  DCM/1 -> "Gravity "/2(DCM)
  Bus Selector4/2 -> "Gravity "/1(g)  "<g>"
  Sum/1 -> Total Force/1  "Ftot"
  Forces and Moments/2(LMN) -> Total Moment/1  "Mtot"
  "Pilot "/1 -> "Engine "/2(Pilot)
  FltParams/1 -> "Engine "/1(Fltparams), Forces and Moments/2(Fltparams), Aerodynamics/2(FltParams)
  Actuators/1(uaero-out) -> Aerodynamics/1(Uaero)
  EnvirBus/1 -> Bus Selector4/1

== system do178b_dhc2_rev_new/DeHavilland Beaver Airframe/Aircraft Dynamics/Total Forces and Moments/Actuators ==
  Pilot : Inport
  Aileron Actuator : aerolibobsolete/Second Order Nonlinear Actuator  wn_fin=10*2*pi  z_fin=0.7  fin_max=15*pi/180  fin_min=-15*pi/180  fin_maxrate=40*pi/180  fin_act_0=uaero0(3)
      settings: SourceProductBaseCode=AE
  Bus Selector2 : BusSelector  OutputSignals=uaero
  Demux : Demux
  Elevator Actuator : aerolibobsolete/Second Order Nonlinear Actuator  wn_fin=10*2*pi  z_fin=0.7  fin_max=20*pi/180  fin_min=-20*pi/180  fin_maxrate=40*pi/180  fin_act_0=uaero0(1)
      settings: SourceProductBaseCode=AE
  Initial inputs for aero : Constant  Value=uaero0
  Mux : Mux
  Rudder Actuator : aerolibobsolete/Second Order Nonlinear Actuator  wn_fin=10*2*pi  z_fin=0.7  fin_max=25*pi/180  fin_min=-25*pi/180  fin_maxrate=40*pi/180  fin_act_0=uaero0(3)
      settings: SourceProductBaseCode=AE
  Sum1 : Sum  Inputs=++|  InputSameDT=on  SaturateOnIntegerOverflow=on  OutDataTypeStr=Inherit: Same as first input
  uaero-out : Outport  VectorParamsAs1DForOutWhenUnconnected=off
  wires:
  Pilot/1 -> Bus Selector2/1
  Initial inputs for aero/1 -> Sum1/1
  Demux/4 -> Mux/4
  Demux/1 -> Elevator Actuator/1
  Demux/2 -> Aileron Actuator/1
  Demux/3 -> Rudder Actuator/1
  Mux/1 -> uaero-out/1
  Sum1/1 -> Demux/1
  Bus Selector2/1 -> Sum1/2  "<uaero>"
  Elevator Actuator/1 -> Mux/1
  Aileron Actuator/1 -> Mux/2
  Rudder Actuator/1 -> Mux/3

== system do178b_dhc2_rev_new/DeHavilland Beaver Airframe/Aircraft Dynamics/Total Forces and Moments/Aerodynamics ==
  Uaero : Inport
  FltParams : Inport  Port=2
  Actuator Increments : Subsystem
  Body Rate Damping : Subsystem
  Bus Selector1 : BusSelector  OutputSignals=alpha,beta
  Bus Selector2 : BusSelector  OutputSignals=V,pqr_tot
  Datum Coefficients : Subsystem
  Sum : Sum  Inputs=+++  SaturateOnIntegerOverflow=on
  Aero Coefficients : Outport  VectorParamsAs1DForOutWhenUnconnected=off
  wires:
  Bus Selector1/2 -> Actuator Increments/2(beta), Datum Coefficients/2(beta)  "<beta>"
  Sum/1 -> Aero Coefficients/1
  Body Rate Damping/1(Coefficients) -> Sum/3
  Datum Coefficients/1(Coefficients) -> Sum/1
  Actuator Increments/1(Coefficients) -> Sum/2
  Bus Selector2/1 -> Body Rate Damping/1(V)  "<V>"
  Bus Selector2/2 -> Body Rate Damping/2(p,q,r)  "<pqr_tot>"
  Uaero/1 -> Actuator Increments/3(Actuator Deflections)
  Bus Selector1/1 -> Actuator Increments/1(alpha), Datum Coefficients/1(alpha)  "<alpha>"
  FltParams/1 -> Bus Selector1/1, Bus Selector2/1

== system do178b_dhc2_rev_new/DeHavilland Beaver Airframe/Aircraft Dynamics/Total Forces and Moments/Engine  ==
  Fltparams : Inport
  Pilot : Inport  Port=2
  rho : Inport  Port=3
  Bus Selector4 : BusSelector  OutputSignals=V,alpha
  eng : Subsystem
  pow : Subsystem
  Engine Coefficients : Outport  VectorParamsAs1DForOutWhenUnconnected=off
  wires:
  Bus Selector4/1 -> pow/3(V)  "<V>"
  rho/1 -> pow/1(rho)
  Bus Selector4/2 -> eng/2(alpha)  "<alpha>"
  eng/1(Cprop) -> Engine Coefficients/1
  Pilot/1 -> pow/2(Pilot)
  pow/1(dpt) -> eng/1(dpt)
  Fltparams/1 -> Bus Selector4/1

== system do178b_dhc2_rev_new/DeHavilland Beaver Airframe/Aircraft Dynamics/Total Forces and Moments/Forces and Moments ==
  Aero Coefficients : Inport
  Fltparams : Inport  Port=2
  Engine Coefficients : Inport  Port=3
  Aerodynamic Forces and Moments : aerolibadyn/Aerodynamic Forces and Moments   inputAxes=Body  outputForceAxes=Body  outputMomentAxes=Body  S=beaver_S  b=beaver_b  cbar=beaver_c
  Bus Selector4 : BusSelector  OutputSignals=Qdyn
  Sum : Sum  Inputs=++|  InputSameDT=on  SaturateOnIntegerOverflow=on  OutDataTypeStr=Inherit: Same as first input
  neglect center of gravity and center of pressure effects : Constant  Value=[0 0 0]
  XYZ : Outport  VectorParamsAs1DForOutWhenUnconnected=off
  LMN : Outport  Port=2  VectorParamsAs1DForOutWhenUnconnected=off
  wires:
  Sum/1 -> Aerodynamic Forces and Moments/1
  Aero Coefficients/1 -> Sum/2
  Engine Coefficients/1 -> Sum/1
  Aerodynamic Forces and Moments/2 -> LMN/1
  Fltparams/1 -> Bus Selector4/1
  Aerodynamic Forces and Moments/1 -> XYZ/1
  neglect center of gravity and center of pressure effects/1 -> Aerodynamic Forces and Moments/3, Aerodynamic Forces and Moments/4
  Bus Selector4/1 -> Aerodynamic Forces and Moments/2  "<Qdyn>"

== system do178b_dhc2_rev_new/DeHavilland Beaver Airframe/Aircraft Dynamics/Total Forces and Moments/Gravity  ==
  g : Inport
  DCM : Inport  Port=2
  Gravity in Earth Axes : Gain  Gain=[0 0 beaver_mass]  SaturateOnIntegerOverflow=on  OutDataTypeStr=Inherit: Same as input  ParamDataTypeStr=Inherit: Same as input
  Inertial to Body : Product  Multiplication=Matrix(*)  InputSameDT=on  SaturateOnIntegerOverflow=on  OutDataTypeStr=Inherit: Same as first input
  Reshape : Reshape  OutputDimensionality=Column vector (2-D)
  Reshape1 : Reshape
  Fgrav : Outport  VectorParamsAs1DForOutWhenUnconnected=off
  wires:
  Inertial to Body/1 -> Reshape1/1
  g/1 -> Gravity in Earth Axes/1
  DCM/1 -> Inertial to Body/1
  Gravity in Earth Axes/1 -> Reshape/1
  Reshape/1 -> Inertial to Body/2
  Reshape1/1 -> Fgrav/1

== system do178b_dhc2_rev_new/DeHavilland Beaver Airframe/Aircraft Dynamics/Total Forces and Moments/Aerodynamics/Actuator Increments ==
  alpha : Inport
  beta : Inport  Port=2
  Actuator Deflections : Inport  Port=3
  Aileron : Subsystem
  Elevator : Subsystem
  Flap : Subsystem
  Rudder : Subsystem
  Sum : Sum  Inputs=++++  InputSameDT=on  SaturateOnIntegerOverflow=on  OutDataTypeStr=Inherit: Same as first input
  Coefficients : Outport  VectorParamsAs1DForOutWhenUnconnected=off
  wires:
  Actuator Deflections/1 -> Flap/2(Actuators), Aileron/2(Actuators), Elevator/1(Actuators), Rudder/2(Actuators)
  alpha/1 -> Flap/1(Alpha), Rudder/1(Alpha), Aileron/1(alpha)
  beta/1 -> Elevator/2(Beta)
  Aileron/1(delCoeff) -> Sum/1
  Elevator/1(delCoeff) -> Sum/2
  Rudder/1(delCoeff) -> Sum/3
  Flap/1(delCoeff) -> Sum/4
  Sum/1 -> Coefficients/1

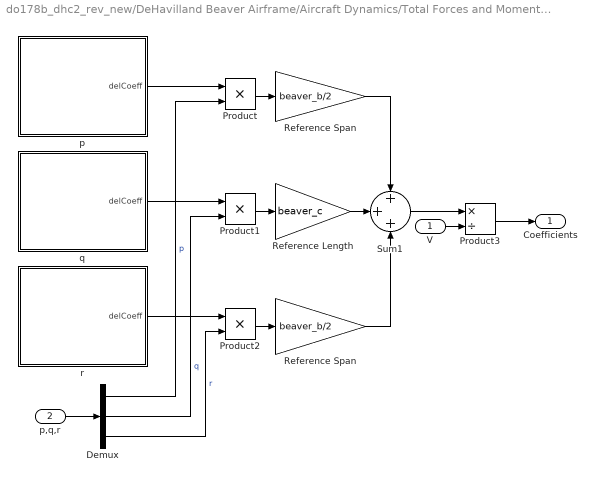
== system do178b_dhc2_rev_new/DeHavilland Beaver Airframe/Aircraft Dynamics/Total Forces and Moments/Aerodynamics/Body Rate Damping ==
  V : Inport
  p,q,r : Inport  Port=2
  Demux : Demux  Outputs=3
      settings: DisplayOption=none
  Product : Product  InputSameDT=on  SaturateOnIntegerOverflow=on  OutDataTypeStr=Inherit: Same as first input
  Product1 : Product  InputSameDT=on  SaturateOnIntegerOverflow=on  OutDataTypeStr=Inherit: Same as first input
  Product2 : Product  InputSameDT=on  SaturateOnIntegerOverflow=on  OutDataTypeStr=Inherit: Same as first input
  Product3 : Product  Inputs=*/  InputSameDT=on  SaturateOnIntegerOverflow=on  OutDataTypeStr=Inherit: Same as first input
  Reference Length : Gain  Gain=beaver_c  SaturateOnIntegerOverflow=on  OutDataTypeStr=Inherit: Same as input  ParamDataTypeStr=Inherit: Same as input
  Reference Span : Gain  Gain=beaver_b/2  SaturateOnIntegerOverflow=on  OutDataTypeStr=Inherit: Same as input  ParamDataTypeStr=Inherit: Same as input
  "Reference Span " : Gain  Gain=beaver_b/2  SaturateOnIntegerOverflow=on  OutDataTypeStr=Inherit: Same as input  ParamDataTypeStr=Inherit: Same as input
  Sum1 : Sum  Inputs=+++  InputSameDT=on  SaturateOnIntegerOverflow=on  OutDataTypeStr=Inherit: Same as first input
  p : Subsystem
  q : Subsystem
  r : Subsystem
  Coefficients : Outport  VectorParamsAs1DForOutWhenUnconnected=off
  wires:
  p/1(delCoeff) -> Product/1
  q/1(delCoeff) -> Product1/1
  p,q,r/1 -> Demux/1
  Demux/1 -> Product/2  "p"
  Demux/2 -> Product1/2  "q"
  Demux/3 -> Product2/2  "r"
  Sum1/1 -> Product3/1
  V/1 -> Product3/2
  Product3/1 -> Coefficients/1
  Product1/1 -> Reference Length/1
  Product2/1 -> "Reference Span "/1
  Product/1 -> Reference Span/1
  r/1(delCoeff) -> Product2/1
  Reference Length/1 -> Sum1/2
  Reference Span/1 -> Sum1/1
  "Reference Span "/1 -> Sum1/3

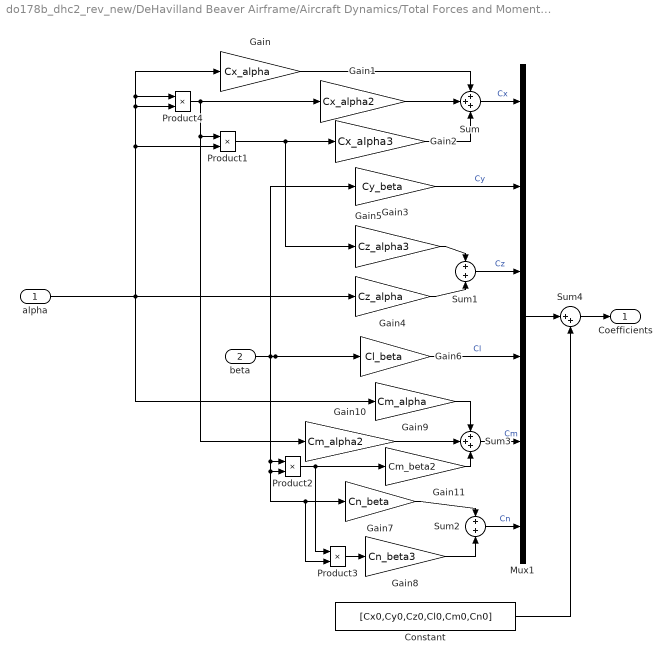
== system do178b_dhc2_rev_new/DeHavilland Beaver Airframe/Aircraft Dynamics/Total Forces and Moments/Aerodynamics/Datum Coefficients ==
  alpha : Inport
  beta : Inport  Port=2
  Constant : Constant  Value=[Cx0,Cy0,Cz0,Cl0,Cm0,Cn0]
  Gain : Gain  Gain=Cx_alpha  SaturateOnIntegerOverflow=on  OutDataTypeStr=Inherit: Same as input  ParamDataTypeStr=Inherit: Same as input
  Gain1 : Gain  Gain=Cx_alpha2  SaturateOnIntegerOverflow=on  OutDataTypeStr=Inherit: Same as input  ParamDataTypeStr=Inherit: Same as input
  Gain10 : Gain  Gain=Cm_alpha2  SaturateOnIntegerOverflow=on  OutDataTypeStr=Inherit: Same as input  ParamDataTypeStr=Inherit: Same as input
  Gain11 : Gain  Gain=Cm_beta2  SaturateOnIntegerOverflow=on  OutDataTypeStr=Inherit: Same as input  ParamDataTypeStr=Inherit: Same as input
  Gain2 : Gain  Gain=Cx_alpha3  SaturateOnIntegerOverflow=on  OutDataTypeStr=Inherit: Same as input  ParamDataTypeStr=Inherit: Same as input
  Gain3 : Gain  Gain=Cy_beta  SaturateOnIntegerOverflow=on  OutDataTypeStr=Inherit: Same as input  ParamDataTypeStr=Inherit: Same as input
  Gain4 : Gain  Gain=Cz_alpha  SaturateOnIntegerOverflow=on  OutDataTypeStr=Inherit: Same as input  ParamDataTypeStr=Inherit: Same as input
  Gain5 : Gain  Gain=Cz_alpha3  SaturateOnIntegerOverflow=on  OutDataTypeStr=Inherit: Same as input  ParamDataTypeStr=Inherit: Same as input
  Gain6 : Gain  Gain=Cl_beta  SaturateOnIntegerOverflow=on  OutDataTypeStr=Inherit: Same as input  ParamDataTypeStr=Inherit: Same as input
  Gain7 : Gain  Gain=Cn_beta  SaturateOnIntegerOverflow=on  OutDataTypeStr=Inherit: Same as input  ParamDataTypeStr=Inherit: Same as input
  Gain8 : Gain  Gain=Cn_beta3  SaturateOnIntegerOverflow=on  OutDataTypeStr=Inherit: Same as input  ParamDataTypeStr=Inherit: Same as input
  Gain9 : Gain  Gain=Cm_alpha  SaturateOnIntegerOverflow=on  OutDataTypeStr=Inherit: Same as input  ParamDataTypeStr=Inherit: Same as input
  Mux1 : Mux  Inputs=6
  Product{1..4} (4 alike) : Product  InputSameDT=on  SaturateOnIntegerOverflow=on  OutDataTypeStr=Inherit: Same as first input
  Sum : Sum  Inputs=+++  SaturateOnIntegerOverflow=on
  Sum1 : Sum  SaturateOnIntegerOverflow=on
  Sum2 : Sum  SaturateOnIntegerOverflow=on
  Sum3 : Sum  Inputs=+++  SaturateOnIntegerOverflow=on
  Sum4 : Sum  Inputs=|++  SaturateOnIntegerOverflow=on
  Coefficients : Outport  VectorParamsAs1DForOutWhenUnconnected=off
  wires:
  Constant/1 -> Sum4/2
  Sum4/1 -> Coefficients/1
  Mux1/1 -> Sum4/1
  Gain10/1 -> Sum3/2
  Product2/1 -> Product3/1, Gain11/1
  Gain11/1 -> Sum3/3
  Gain9/1 -> Sum3/1
  Sum3/1 -> Mux1/5  "Cm"
  Product3/1 -> Gain8/1
  Gain8/1 -> Sum2/2
  Gain7/1 -> Sum2/1
  Gain5/1 -> Sum1/1
  Gain4/1 -> Sum1/2
  Product1/1 -> Gain5/1, Gain2/1
  Gain2/1 -> Sum/3
  Product4/1 -> Product1/1, Gain10/1, Gain1/1
  Gain1/1 -> Sum/2
  Gain/1 -> Sum/1
  Sum2/1 -> Mux1/6  "Cn"
  Sum/1 -> Mux1/1  "Cx"
  Sum1/1 -> Mux1/3  "Cz"
  Gain3/1 -> Mux1/2  "Cy"
  Gain6/1 -> Mux1/4  "Cl"
  alpha/1 -> Product1/2, Product4/2, Product4/1, Gain/1, Gain9/1, Gain4/1
  beta/1 -> Gain3/1, Product3/2, Gain7/1, Product2/2, Product2/1, Gain6/1

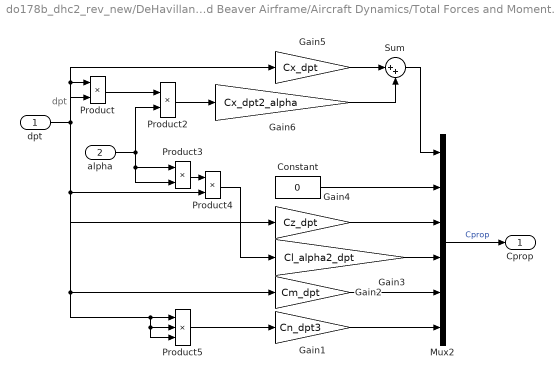
== system do178b_dhc2_rev_new/DeHavilland Beaver Airframe/Aircraft Dynamics/Total Forces and Moments/Engine /eng ==
  note: dpt
  dpt : Inport
  alpha : Inport  Port=2
  Constant : Constant  Value=0
  Gain1 : Gain  Gain=Cn_dpt3  SaturateOnIntegerOverflow=on  OutDataTypeStr=Inherit: Same as input  ParamDataTypeStr=Inherit: Same as input
  Gain2 : Gain  Gain=Cm_dpt  SaturateOnIntegerOverflow=on  OutDataTypeStr=Inherit: Same as input  ParamDataTypeStr=Inherit: Same as input
  Gain3 : Gain  Gain=Cl_alpha2_dpt  SaturateOnIntegerOverflow=on  OutDataTypeStr=Inherit: Same as input  ParamDataTypeStr=Inherit: Same as input
  Gain4 : Gain  Gain=Cz_dpt  SaturateOnIntegerOverflow=on  OutDataTypeStr=Inherit: Same as input  ParamDataTypeStr=Inherit: Same as input
  Gain5 : Gain  Gain=Cx_dpt  SaturateOnIntegerOverflow=on  OutDataTypeStr=Inherit: Same as input  ParamDataTypeStr=Inherit: Same as input
  Gain6 : Gain  Gain=Cx_dpt2_alpha  SaturateOnIntegerOverflow=on  OutDataTypeStr=Inherit: Same as input  ParamDataTypeStr=Inherit: Same as input
  Mux2 : Mux  Inputs=6
  Product{,2..4} (4 alike) : Product  SaturateOnIntegerOverflow=on  OutDataTypeStr=Inherit: Same as first input
  Product5 : Product  Inputs=3  SaturateOnIntegerOverflow=on  OutDataTypeStr=Inherit: Same as first input
  Sum : Sum  Inputs=|++  SaturateOnIntegerOverflow=on
  Cprop : Outport  VectorParamsAs1DForOutWhenUnconnected=off
  wires:
  Product5/1 -> Gain1/1
  Sum/1 -> Mux2/1
  Gain6/1 -> Sum/2
  Gain5/1 -> Sum/1
  Constant/1 -> Mux2/2
  Gain4/1 -> Mux2/3
  Gain3/1 -> Mux2/4
  Gain2/1 -> Mux2/5
  Gain1/1 -> Mux2/6
  Product4/1 -> Gain3/1
  Product2/1 -> Gain6/1
  dpt/1 -> Gain5/1, Product5/3, Product5/2, Product5/1, Gain2/1, Gain4/1, Product/2, Product/1, Product4/2
  alpha/1 -> Product2/2, Product3/1, Product3/2
  Mux2/1 -> Cprop/1  "Cprop"
  Product/1 -> Product2/1
  Product3/1 -> Product4/1

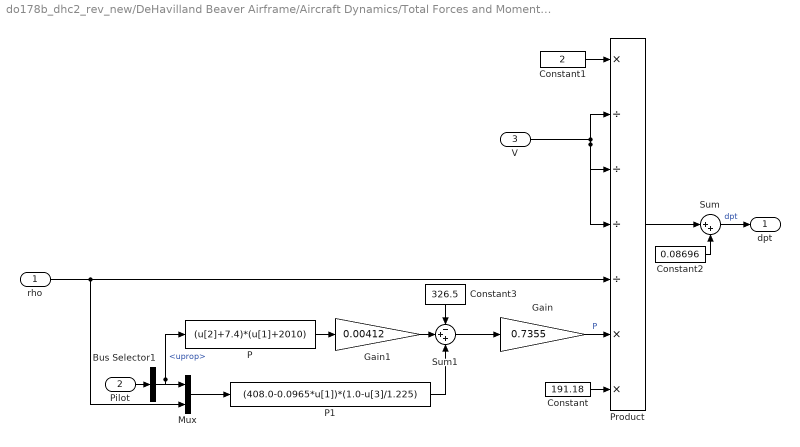
== system do178b_dhc2_rev_new/DeHavilland Beaver Airframe/Aircraft Dynamics/Total Forces and Moments/Engine /pow ==
  rho : Inport
  Pilot : Inport  Port=2
  V : Inport  Port=3
  Bus Selector1 : BusSelector  OutputSignals=uprop
  Constant : Constant  Value=191.18
  Constant1 : Constant  Value=2
  Constant2 : Constant  Value=0.08696
  Constant3 : Constant  Value=326.5
  Gain : Gain  Gain=0.7355  SaturateOnIntegerOverflow=on  OutDataTypeStr=Inherit: Same as input  ParamDataTypeStr=Inherit: Same as input
  Gain1 : Gain  Gain=0.00412  SaturateOnIntegerOverflow=on  OutDataTypeStr=Inherit: Same as input  ParamDataTypeStr=Inherit: Same as input
  Mux : Mux  Inputs=2
  P : Fcn  Expr=(u[2]+7.4)*(u[1]+2010)
  P1 : Fcn  Expr=(408.0-0.0965*u[1])*(1.0-u[3]/1.225)
  Product : Product  Inputs=*////**  SaturateOnIntegerOverflow=on  OutDataTypeStr=Inherit: Same as first input
  Sum : Sum  Inputs=|++  SaturateOnIntegerOverflow=on
  Sum1 : Sum  Inputs=-++  SaturateOnIntegerOverflow=on
  dpt : Outport  VectorParamsAs1DForOutWhenUnconnected=off
  wires:
  P1/1 -> Sum1/3
  Constant3/1 -> Sum1/1
  Gain1/1 -> Sum1/2
  Mux/1 -> P1/1
  Sum1/1 -> Gain/1
  P/1 -> Gain1/1
  Gain/1 -> Product/6  "P"
  rho/1 -> Mux/2, Product/5
  Sum/1 -> dpt/1  "dpt"
  V/1 -> Product/4, Product/3, Product/2
  Bus Selector1/1 -> Mux/1, P/1  "<uprop>"
  Constant/1 -> Product/7
  Constant1/1 -> Product/1
  Product/1 -> Sum/1
  Constant2/1 -> Sum/2
  Pilot/1 -> Bus Selector1/1

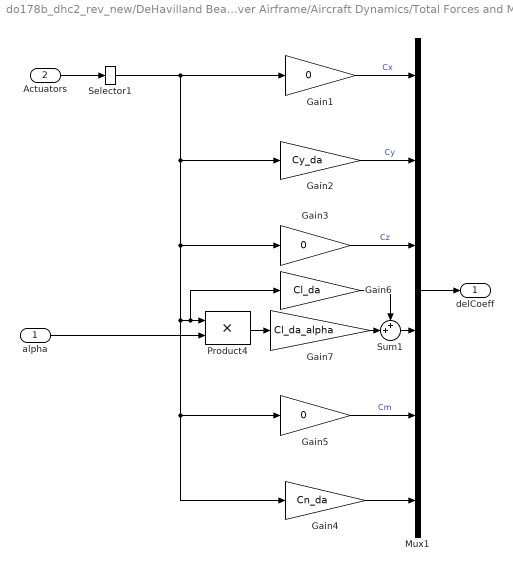
== system do178b_dhc2_rev_new/DeHavilland Beaver Airframe/Aircraft Dynamics/Total Forces and Moments/Aerodynamics/Actuator Increments/Aileron ==
  alpha : Inport
  Actuators : Inport  Port=2
  Gain1 : Gain  Gain=0  SaturateOnIntegerOverflow=on  OutDataTypeStr=Inherit: Same as input  ParamDataTypeStr=Inherit: Same as input
  Gain2 : Gain  Gain=Cy_da  SaturateOnIntegerOverflow=on  OutDataTypeStr=Inherit: Same as input  ParamDataTypeStr=Inherit: Same as input
  Gain3 : Gain  Gain=0  SaturateOnIntegerOverflow=on  OutDataTypeStr=Inherit: Same as input  ParamDataTypeStr=Inherit: Same as input
  Gain4 : Gain  Gain=Cn_da  SaturateOnIntegerOverflow=on  OutDataTypeStr=Inherit: Same as input  ParamDataTypeStr=Inherit: Same as input
  Gain5 : Gain  Gain=0  SaturateOnIntegerOverflow=on  OutDataTypeStr=Inherit: Same as input  ParamDataTypeStr=Inherit: Same as input
  Gain6 : Gain  Gain=Cl_da  SaturateOnIntegerOverflow=on  OutDataTypeStr=Inherit: Same as input  ParamDataTypeStr=Inherit: Same as input
  Gain7 : Gain  Gain=Cl_da_alpha  SaturateOnIntegerOverflow=on  OutDataTypeStr=Inherit: Same as input  ParamDataTypeStr=Inherit: Same as input
  Mux1 : Mux  Inputs=6
  Product4 : Product  InputSameDT=on  SaturateOnIntegerOverflow=on  OutDataTypeStr=Inherit: Same as first input
  Selector1 : Selector  InputPortWidth=4  IndexOptions=Index vector (dialog)  Indices=2  OutputSizes=1
  Sum1 : Sum  Inputs=++|  SaturateOnIntegerOverflow=on
  delCoeff : Outport  VectorParamsAs1DForOutWhenUnconnected=off
  wires:
  Gain6/1 -> Sum1/1
  Sum1/1 -> Mux1/4
  Gain7/1 -> Sum1/2
  Product4/1 -> Gain7/1
  Gain1/1 -> Mux1/1  "Cx"
  alpha/1 -> Product4/2
  Actuators/1 -> Selector1/1
  Mux1/1 -> delCoeff/1
  Gain2/1 -> Mux1/2  "Cy"
  Gain3/1 -> Mux1/3  "Cz"
  Gain5/1 -> Mux1/5  "Cm"
  Gain4/1 -> Mux1/6
  Selector1/1 -> Gain1/1, Gain2/1, Gain3/1, Gain6/1, Product4/1, Gain5/1, Gain4/1

== system do178b_dhc2_rev_new/DeHavilland Beaver Airframe/Aircraft Dynamics/Total Forces and Moments/Aerodynamics/Actuator Increments/Elevator ==
  Actuators : Inport
  Beta : Inport  Port=2
  Constant1 : Constant  Value=0
  Gain1 : Gain  Gain=Cz_de  SaturateOnIntegerOverflow=on  OutDataTypeStr=Inherit: Same as input  ParamDataTypeStr=Inherit: Same as input
  Gain2 : Gain  Gain=Cz_de_beta  SaturateOnIntegerOverflow=on  OutDataTypeStr=Inherit: Same as input  ParamDataTypeStr=Inherit: Same as input
  Gain3 : Gain  Gain=Cm_de  SaturateOnIntegerOverflow=on  OutDataTypeStr=Inherit: Same as input  ParamDataTypeStr=Inherit: Same as input
  Mux1 : Mux  Inputs=6
  Product4 : Product  Inputs=3  InputSameDT=on  SaturateOnIntegerOverflow=on  OutDataTypeStr=Inherit: Same as first input
  Selector1 : Selector  InputPortWidth=4  IndexOptions=Index vector (dialog)  Indices=1  OutputSizes=1
  Sum1 : Sum  SaturateOnIntegerOverflow=on
  delCoeff : Outport  VectorParamsAs1DForOutWhenUnconnected=off
  wires:
  Gain3/1 -> Mux1/5
  Gain1/1 -> Sum1/2
  Gain2/1 -> Sum1/1
  Sum1/1 -> Mux1/3
  Product4/1 -> Gain2/1
  Beta/1 -> Product4/2, Product4/1
  Mux1/1 -> delCoeff/1
  Selector1/1 -> Gain3/1, Gain1/1, Product4/3
  Constant1/1 -> Mux1/1, Mux1/2, Mux1/4, Mux1/6
  Actuators/1 -> Selector1/1

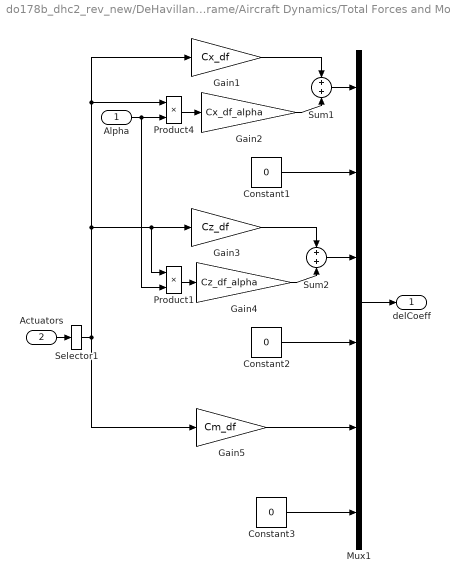
== system do178b_dhc2_rev_new/DeHavilland Beaver Airframe/Aircraft Dynamics/Total Forces and Moments/Aerodynamics/Actuator Increments/Flap ==
  Alpha : Inport
  Actuators : Inport  Port=2
  Constant1 : Constant  Value=0
  Constant2 : Constant  Value=0
  Constant3 : Constant  Value=0
  Gain1 : Gain  Gain=Cx_df  SaturateOnIntegerOverflow=on  OutDataTypeStr=Inherit: Same as input  ParamDataTypeStr=Inherit: Same as input
  Gain2 : Gain  Gain=Cx_df_alpha  SaturateOnIntegerOverflow=on  OutDataTypeStr=Inherit: Same as input  ParamDataTypeStr=Inherit: Same as input
  Gain3 : Gain  Gain=Cz_df  SaturateOnIntegerOverflow=on  OutDataTypeStr=Inherit: Same as input  ParamDataTypeStr=Inherit: Same as input
  Gain4 : Gain  Gain=Cz_df_alpha  SaturateOnIntegerOverflow=on  OutDataTypeStr=Inherit: Same as input  ParamDataTypeStr=Inherit: Same as input
  Gain5 : Gain  Gain=Cm_df  SaturateOnIntegerOverflow=on  OutDataTypeStr=Inherit: Same as input  ParamDataTypeStr=Inherit: Same as input
  Mux1 : Mux  Inputs=6
  Product1 : Product  InputSameDT=on  SaturateOnIntegerOverflow=on  OutDataTypeStr=Inherit: Same as first input
  Product4 : Product  InputSameDT=on  SaturateOnIntegerOverflow=on  OutDataTypeStr=Inherit: Same as first input
  Selector1 : Selector  InputPortWidth=4  IndexOptions=Index vector (dialog)  Indices=4  OutputSizes=1
  Sum1 : Sum  SaturateOnIntegerOverflow=on
  Sum2 : Sum  SaturateOnIntegerOverflow=on
  delCoeff : Outport  VectorParamsAs1DForOutWhenUnconnected=off
  wires:
  Selector1/1 -> Gain1/1, Product4/1, Product1/1, Gain3/1, Gain5/1
  Actuators/1 -> Selector1/1
  Gain5/1 -> Mux1/5
  Gain3/1 -> Sum2/1
  Gain4/1 -> Sum2/2
  Product1/1 -> Gain4/1
  Gain1/1 -> Sum1/1
  Gain2/1 -> Sum1/2
  Product4/1 -> Gain2/1
  Alpha/1 -> Product1/2, Product4/2
  Mux1/1 -> delCoeff/1
  Sum1/1 -> Mux1/1
  Sum2/1 -> Mux1/3
  Constant1/1 -> Mux1/2
  Constant2/1 -> Mux1/4
  Constant3/1 -> Mux1/6
